simulink model "Multifil"  (Simulink 3.00)
settings: Solver=ode45  StartTime=0.0  StopTime=10.0  RelTol=1e-3
libraries: Dequiv x4, simulink_extras x2, simulink3 x1
settings Model: LastModifiedBy=campa

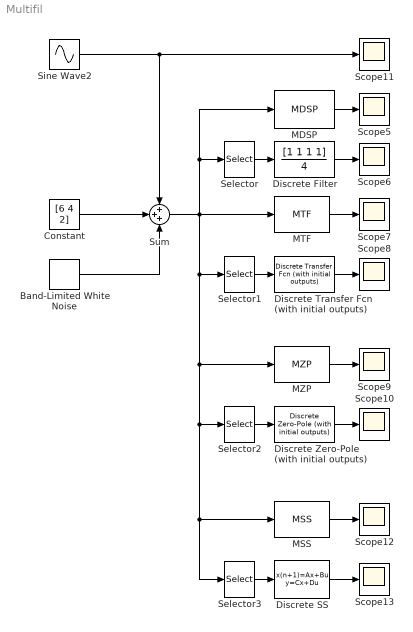
== system Multifil ==
  Band-Limited White Noise : simulink3/Sources/Band-Limited White Noise  Cov=0.001*ones(3,1)  Ts=0.025  seed=[1 2 3]
  Constant : Constant  Value=[6 4 2]
  Discrete Transfer Fcn (with initial outputs) : simulink_extras/Additional Discrete/Discrete Transfer Fcn (with initial outputs)  N=[1 1 1 1]  D=[4 0 0 0]  U0=6  Y0=6  TS=0.025
  Discrete Zero-Pole (with initial outputs) : simulink_extras/Additional Discrete/Discrete Zero-Pole (with initial outputs)  Z=[-1 sqrt(-1) -sqrt(-1)]  P=[0 0 0]  K=1/4  U0=6  Y0=6  TS=0.025
  Discrete Filter : DiscreteFilter  Numerator=[1 1 1 1]  Denominator=4  SampleTime=0.025
  Discrete SS : DiscreteStateSpace  A=diag(ones(1,3-1),1)  B=[0;0;1]  C=[1 1 1]/4  D=1/4  X0=[6;6;6]  SampleTime=0.025
  MDSP : Dequiv/MDSP  ni=3  num=[1 1 1 1]  den=4  u0=[6 4 2]'  T=0.025
  MSS : Dequiv/MSS  n=3  a=diag(ones(1,3-1),1)  b=[0;0;1]  c=[1 1 1]/4  d=1/4  u0=[6 4 2]'  T=0.025
  MTF : Dequiv/MTF  ni=3  num=[1 1 1 1]  den=[4 0 0 0]  u0=[6 4 2]'  T=0.025
  MZP : Dequiv/MZP  ni=3  Z=[-1 sqrt(-1) -sqrt(-1)]  P=[0 0 0]  K=1/4  u0=[6 4 2]'  T=0.025
  Scope{5..13} (9 alike) : Scope
      Scope10 settings: TimeRange=10  YMin=-2  YMax=10  SaveToWorkspace=off  SaveName=ScopeData
      Scope11 settings: TimeRange=10  YMin=-1  YMax=1  SaveToWorkspace=off  SaveName=ScopeData
      Scope12 settings: TimeRange=10  YMin=-2  YMax=10  SaveToWorkspace=off  SaveName=ScopeData
      Scope13 settings: TimeRange=10  YMin=-2  YMax=10  SaveToWorkspace=off  SaveName=ScopeData
      Scope5 settings: TimeRange=10  YMin=-2  YMax=10  SaveToWorkspace=off  SaveName=ScopeData
      Scope6 settings: TimeRange=10  YMin=-2  YMax=10  SaveToWorkspace=off  SaveName=ScopeData
      Scope7 settings: TimeRange=10  YMin=-2  YMax=10  SaveToWorkspace=off  SaveName=ScopeData
      Scope8 settings: TimeRange=10  YMin=-2  YMax=10  SaveToWorkspace=off  SaveName=ScopeData
      Scope9 settings: TimeRange=10  YMin=-2  YMax=10  SaveToWorkspace=off  SaveName=ScopeData
  Selector{,1..3} (4 alike) : Selector  Elements=1  InputPortWidth=3
  Sine Wave2 : Sin  Amplitude=1  Frequency=1.5  Phase=0  SampleTime=0
  Sum : Sum  Inputs=+++  SaturateOnIntegerOverflow=on
  wires:
  Sum/1 -> MTF/1, Selector1/1, MZP/1, Selector2/1, MSS/1, Selector3/1, MDSP/1, Selector/1
  Band-Limited White Noise/1 -> Sum/3
  Constant/1 -> Sum/2
  MDSP/1 -> Scope5/1
  Sine Wave2/1 -> Sum/1, Scope11/1
  Discrete Filter/1 -> Scope6/1
  Selector/1 -> Discrete Filter/1
  MTF/1 -> Scope7/1
  Selector1/1 -> Discrete Transfer Fcn (with initial outputs)/1
  Discrete Transfer Fcn (with initial outputs)/1 -> Scope8/1
  MSS/1 -> Scope12/1
  Selector3/1 -> Discrete SS/1
  Discrete SS/1 -> Scope13/1
  Discrete Zero-Pole (with initial outputs)/1 -> Scope10/1
  Selector2/1 -> Discrete Zero-Pole (with initial outputs)/1
  MZP/1 -> Scope9/1
